simulink model "LH2Ship_Simulink_Winter"  (R2018b)
settings: Solver=VariableStepAuto  StartTime=0.0  StopTime=3600*24*7  FixedStep=0.1  MaxStep=0.5  MinStep=0.001  RelTol=1e-7  AbsTol=1e-7
values from neighbouring files (symbols this model uses):
  BoilerEff = 0.85    [PEMFC_Model.m]
  H2Consumption_kg = H2SupplyMolRate(:,1:iPmaxtot).*H2_kg_mol    [PEMFC_Model.m]
  H2Exhaust_kg = H2ExhaustMolRate(:,1:iPmaxtot).*H2_kg_mol    [PEMFC_Model.m]
  H2hhv = 141.7*10^6    (= 141700000)    [PEMFC_Model.m]
  H2lhv = 119.96*10^6    (= 119960000)    [PEMFC_Model.m]
  H2u = (0.05:0.1:0.95)    [PEMFC_Model.m]
  HeatStorageCapacity = 4.5e10    (= 45000000000)    [PEMFC_Model.m]
  HeatStorageEff = 0.9    [PEMFC_Model.m]
  HeatStorageIC = 1    [PEMFC_Model.m]
  i_FC = iCell(1,1:iPmaxtot)    [PEMFC_Model.m]
  Nstacks = 330    [PEMFC_Model.m]
  PowerElectronicsEff = 0.9    [PEMFC_Model.m]
  RecoveredHeat = NetHeatOut(:,1:iPmaxtot)    [PEMFC_Model.m]
  V_FC = Vout(:,1:iPmaxtot)    [PEMFC_Model.m]
undefined symbols (not defined in the file or in its folder): BatteryCapacity, BattInitialSOC, mass, Rt, v, VDCBus
libraries: fl_lib x14, nesl_utility x13, simulink x6, pe_lib x2
settings Model: SimulationMode=accelerator  Creator=age  LastModifiedBy=alber
settings SolverCC: InitialStep=0.001  MaxConsecutiveMinStep=2  ZeroCrossControl=DisableAll
settings DataIOCC: LimitDataPoints=on  MaxDataPoints=10000
settings OptimizationCC: LifeSpan=inf
settings DebuggingCC: AllowSymbolicDim=off  LibraryContextMissingDiagnostic=none  SFUnexpectedBacktrackingDiag=warning  SFNoUnconditionalDefaultTransitionDiag=warning  SFExecutionAtInitializationDiag=none
settings SFSimCC: SimUseLocalCustomCode=off
settings RTWCC: RTWUseLocalCustomCode=off
settings CodeAppCC: StateflowObjectComments=on
settings GRTTargetCC: TargetLangStandard=C89/C90 (ANSI)  GeneratePreprocessorConditionals=Disable all
settings ConfigComp: CovMetricSettings=dw  CovHtmlReporting=on  CovSaveCumulativeToWorkspaceVar=on  CovSaveSingleToWorkspaceVar=on  CovExternalEMLEnable=off  CovSFcnEnable=off
settings SimscapeCC: SimscapeLogLimitData=off  SimscapeLogDataHistory=10000

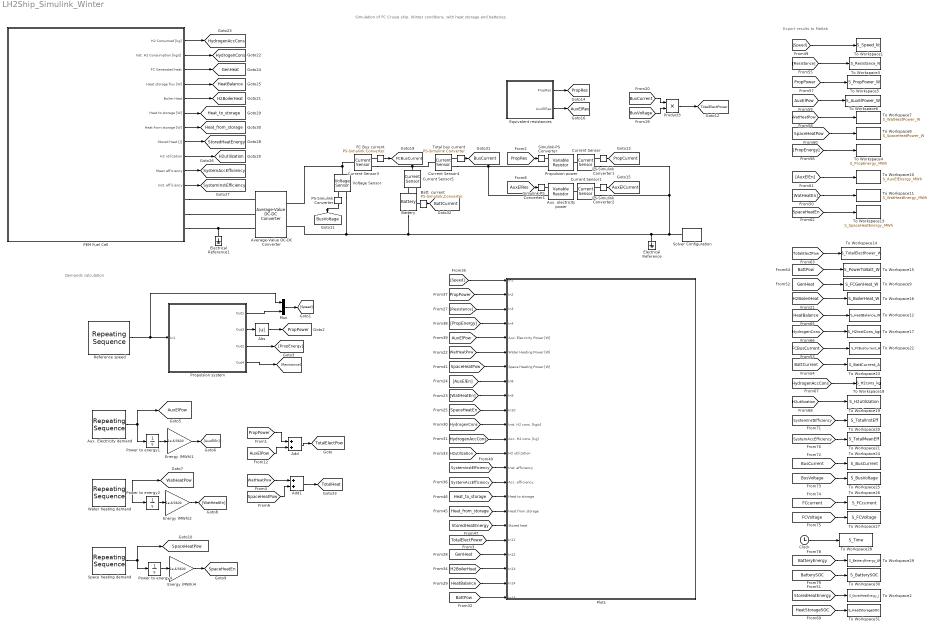
== system LH2Ship_Simulink_Winter ==
  note: Demands calculation
  note: Export results to Matlab
  note: Simulation of FC Cruise ship.
      | Winter conditions, with heat storage and batteries.
  Abs : Abs
  Add : Sum
  Add1 : Sum
  Aux. Electricity demand : simulink/Sources/Repeating Sequence  rep_seq_t=AuxElectProfile.t  rep_seq_y=AuxElectProfile.Elect  mask(Repeating table){}
      mask Display: image('RefSpeed.PNG');
  Aux. electricity power : fl_lib/Electrical/Electrical Elements/Variable Resistor  Rmin=2.8571e-4 Ohm  i_specify=off  i_priority=None  i=0 A  i_nominal_specify=off  i_nominal_unit=A  i_nominal_value=1  v_specify=off  v_priority=None  v=0 V  v_nominal_specify=off  v_nominal_unit=V  v_nominal_value=1
  Average-Value DC-DC Converter : pe_lib/Semiconductors/Average-Value DC-DC Converter  converter_type=3
      settings: SourceProductName=Simscape Power Systems  SourceProductBaseCode=PS
  Batt. current : nesl_utility/PS-Simulink Converter  PhysicalDomain=network_engine_domain  SubClassName=ps_output  LeftPortType=input  RightPortType=output  PseudoPeriodic=off  Frequencies=[]  Unit=1  AffineConversion=off
  Battery : pe_lib/Sources/Battery  Vnom=100 V  R1=0.00016667 Ohm  prm_AH=1  AH=6000 hr*A  V1=75 V  AH1=5426.087 hr*A  prm_R2=1  R2=2000 Ohm  prm_dyn=1  Rp1=0.0005 Ohm  tau1=10 s  Rp2=0.005 Ohm  tau2=30 s  Rp3=0.005 Ohm  tau3=30 s  Rp4=0.005 Ohm  tau4=30 s  Rp5=0.005 Ohm  tau5=30 s  prm_fade=1  N_fade=100  AH_fade=45 hr*A  R1_fade=2.02 Ohm  V1_fade=10.35 V  i_specify=on  i_priority=Low  i=0 A  i_nominal_specify=off  i_nominal_unit=A  i_nominal_value=1  v_specify=on  v_priority=None  v=100 V  v_nominal_specify=off  v_nominal_unit=V  v_nominal_value=1  charge_specify=on  charge_priority=High  charge=3000 hr*A  charge_nominal_specify=off  charge_nominal_unit=hr*A  charge_nominal_value=1  num_cycles_specify=on  num_cycles_priority=None  num_cycles=0  num_cycles_nominal_specify=off  num_cycles_nominal_unit=1  num_cycles_nominal_value=1  thermal_mass=30000 J/K  Tmeas=298.15 K  Vnom_T2=12 V  R1_T2=2.2 Ohm  V1_T2=11.4 V  R2_T2=2200 Ohm  Rp1_T2=0.005 Ohm  tau1_T2=30 s  Rp2_T2=0.005 Ohm  tau2_T2=30 s  Rp3_T2=0.005 Ohm  tau3_T2=30 s  Rp4_T2=0.005 Ohm  tau4_T2=30 s  Rp5_T2=0.005 Ohm  tau5_T2=30 s  Tmeas2=273.15 K  temperature_specify=off  temperature_priority=High  temperature=298.15 K  temperature_nominal_specify=off  temperature_nominal_unit=K  temperature_nominal_value=1
      settings: SourceProductName=Simscape Power Systems  SourceProductBaseCode=PS
  Clock : Clock
  Current Sensor{,1,3..5} (5 alike) : fl_lib/Electrical/Electrical Sensors/Current Sensor
  Electrical Reference : fl_lib/Electrical/Electrical Elements/Electrical Reference
      settings: SourceProductName=Foundation Library
  Electrical Reference1 : fl_lib/Electrical/Electrical Elements/Electrical Reference
      settings: SourceProductName=Foundation Library
  Energy (MWh)1 : Gain  Gain=1e-6/3600
  Energy (MWh)2 : Gain  Gain=1e-6/3600
  Energy (MWh)4 : Gain  Gain=1e-6/3600
  Equivalent resistances : Subsystem
  FC Bus current : nesl_utility/PS-Simulink Converter  PhysicalDomain=network_engine_domain  SubClassName=ps_output  LeftPortType=input  RightPortType=output  PseudoPeriodic=off  Frequencies=[]  Unit=1  AffineConversion=off
  Mux : Mux  Inputs=2
  PEM Fuel Cell : Subsystem
  PS-Simulink Converter : nesl_utility/PS-Simulink Converter  PhysicalDomain=network_engine_domain  SubClassName=ps_output  LeftPortType=input  RightPortType=output  PseudoPeriodic=off  Frequencies=[]  Unit=1  AffineConversion=off
  PS-Simulink Converter1 : nesl_utility/PS-Simulink Converter  PhysicalDomain=network_engine_domain  SubClassName=ps_output  LeftPortType=input  RightPortType=output  PseudoPeriodic=off  Frequencies=[]  Unit=1  AffineConversion=off
  PS-Simulink Converter2 : nesl_utility/PS-Simulink Converter  PhysicalDomain=network_engine_domain  SubClassName=ps_output  LeftPortType=input  RightPortType=output  PseudoPeriodic=off  Frequencies=[]  Unit=1  AffineConversion=off
  Plots : Subsystem
  Power to energy1 : Integrator  LowerSaturationLimit=0
  Power to energy2 : Integrator  LowerSaturationLimit=0
  Power to energy4 : Integrator  LowerSaturationLimit=0
  Product3 : Product
  Propulsion power : fl_lib/Electrical/Electrical Elements/Variable Resistor  Rmin=2.8571e-4 Ohm  i_specify=off  i_priority=None  i=0 A  i_nominal_specify=off  i_nominal_unit=A  i_nominal_value=1  v_specify=off  v_priority=None  v=0 V  v_nominal_specify=off  v_nominal_unit=V  v_nominal_value=1
  Propulsion system : Subsystem
  Reference speed : simulink/Sources/Repeating Sequence  rep_seq_t=SpeedProfile.Time  rep_seq_y=SpeedProfile.Speed  mask(Repeating table){}
      mask Display: image('RefSpeed.PNG');
  Simulink-PS Converter : nesl_utility/Simulink-PS Converter  PhysicalDomain=network_engine_domain  SubClassName=ps_input  LeftPortType=input  RightPortType=output  PseudoPeriodic=off  Frequencies=[]  NoiseDistribution=none  NoiseParameters=[]  Unit=1  AffineConversion=off  FilteringAndDerivatives=provide  SimscapeFilterOrder=1  InputFilterTimeConstant=0.001  UdotUserProvided=0
  Simulink-PS Converter1 : nesl_utility/Simulink-PS Converter  PhysicalDomain=network_engine_domain  SubClassName=ps_input  LeftPortType=input  RightPortType=output  PseudoPeriodic=off  Frequencies=[]  NoiseDistribution=none  NoiseParameters=[]  Unit=1  AffineConversion=off  FilteringAndDerivatives=provide  SimscapeFilterOrder=1  InputFilterTimeConstant=0.001  UdotUserProvided=0
  Solver Configuration : nesl_utility/Solver Configuration  PhysicalDomain=network_engine_domain  SubClassName=solver  LeftPortType=input  RightPortType=generic  Tones=[]  Harmonics=[]  SimulateNoise=off  Profile=off  UseLocalSampling=off  EnableSwitchedLinearOptims=on  FrequencyDomain=off  UseCCode=off  RelTol=0.001  AbsTol=1e-06  MinStep=1e-09  ToWorkspace=off  RevertToSquareIcSolve=off  NumHomotopyIterations=100  PhasorMode=off  PhasorModeNumHarmonics=1  DoDC=on  ResidualTolerance=1e-09  UseLocalSolver=off  LocalSolverChoice=NE_BACKWARD_EULER_ADVANCER  LocalSolverSampleTime=0.001  DoFixedCost=off  MaxNonlinIter=3  MaxModeIter=2  LinearAlgebra=auto  EquationFormulation=NE_TIME_EF  DelaysMemoryBudget=1024  AutomaticFiltering=on  FilteringTimeConstant=0.001  PartitionStorageMethod=AS_NEEDED  PartitionMemoryBudget=1024
  Space heating demand : simulink/Sources/Repeating Sequence  rep_seq_t=SpaceHeatingProfile_Winter.t  rep_seq_y=SpaceHeatingProfile_Winter.Heat  mask(Repeating table){}
      mask Display: image('RefSpeed.PNG');
  To Workspace1 : ToWorkspace  VariableName=S_Speed_kt  SampleTime=30
  To Workspace10 : ToWorkspace  VariableName=S_AuxElEnergy_MWh  SampleTime=30
  To Workspace11 : ToWorkspace  VariableName=S_WatHeatEnergy_MWh  SampleTime=30
  To Workspace12 : ToWorkspace  VariableName=S_HeatBalance_W  SampleTime=30
  To Workspace13 : ToWorkspace  VariableName=S_SpaceHeatEnergy_MWh  SampleTime=30
  To Workspace14 : ToWorkspace  VariableName=S_TotalElectPower_W  SampleTime=30
  To Workspace15 : ToWorkspace  VariableName=S_PowerToBatt_W  SampleTime=30
  To Workspace16 : ToWorkspace  VariableName=S_BoilerHeat_W  SampleTime=30
  To Workspace17 : ToWorkspace  VariableName=S_H2instCons_kgs  SampleTime=30
  To Workspace18 : ToWorkspace  VariableName=S_H2cons_kg  SampleTime=30
  To Workspace19 : ToWorkspace  VariableName=S_H2utilization  SampleTime=30
  To Workspace2 : ToWorkspace  VariableName=S_StoredHeatEnergy_J  SampleTime=30
  To Workspace20 : ToWorkspace  VariableName=S_TotalInstEff  SampleTime=30
  To Workspace21 : ToWorkspace  VariableName=S_TotalMeanEff  SampleTime=30
  To Workspace22 : ToWorkspace  VariableName=S_FCBusCurrent_A  SampleTime=30
  To Workspace23 : ToWorkspace  VariableName=S_BattCurrent_A  SampleTime=30
  To Workspace24 : ToWorkspace  VariableName=S_BusCurrent  SampleTime=30
  To Workspace25 : ToWorkspace  VariableName=S_BusVoltage  SampleTime=30
  To Workspace26 : ToWorkspace  VariableName=S_FCcurrent  SampleTime=30
  To Workspace27 : ToWorkspace  VariableName=S_FCVoltage  SampleTime=30
  To Workspace28 : ToWorkspace  VariableName=S_Time  SampleTime=30
  To Workspace29 : ToWorkspace  VariableName=S_BatteryEnergy_Ah  SampleTime=30
  To Workspace3 : ToWorkspace  VariableName=S_Resistance_N  SampleTime=30
  To Workspace30 : ToWorkspace  VariableName=S_BatterySOC  SampleTime=30
  To Workspace31 : ToWorkspace  VariableName=S_HeatStorageSOC  SampleTime=30
  To Workspace4 : ToWorkspace  VariableName=S_PropEnergy_MWh  SampleTime=30
  To Workspace5 : ToWorkspace  VariableName=S_PropPower_W  SampleTime=30
  To Workspace6 : ToWorkspace  VariableName=S_AuxElPower_W  SampleTime=30
  To Workspace7 : ToWorkspace  VariableName=S_WatHeatPower_W  SampleTime=30
  To Workspace8 : ToWorkspace  VariableName=S_SpaceHeatPower_W  SampleTime=30
  To Workspace9 : ToWorkspace  VariableName=S_FCGenHeat_W  SampleTime=30
  Total bus current : nesl_utility/PS-Simulink Converter  PhysicalDomain=network_engine_domain  SubClassName=ps_output  LeftPortType=input  RightPortType=output  PseudoPeriodic=off  Frequencies=[]  Unit=1  AffineConversion=off
  Voltage Sensor : fl_lib/Electrical/Electrical Sensors/Voltage Sensor
  Water heating demand : simulink/Sources/Repeating Sequence  rep_seq_t=WaterHeatingProfile.t  rep_seq_y=WaterHeatingProfile.Heat  mask(Repeating table){}
      mask Display: image('RefSpeed.PNG');
  tag scope: AuxElCurrent=global, AuxElPow=global, AuxElRes=global, BattCurrent=global, BusCurrent=global, BusVoltage=global, FCBusCurrent=global, GenHeat=global, H2BoilerHeat=global, H2utilization=global, HeatBalance=global, Heat_from_storage=global, Heat_to_storage=global, HydrogenAccCons=global, HydrogenCons=global, PropCurrent=global, PropPower=global, PropRes=global, SpaceHeatEn=global, SpaceHeatPow=global, StoredHeatEnergy=global, SystemAccEfficiency=global, SystemInstEfficiency=global, TotalElectPow=global, TotalElectPower=global, TotalHeat=global, WatHeatPow=global
  wires:
  Power to energy1/1 -> Energy (MWh)1/1
  Propulsion system/4(Out4) -> [Resistance]
  Water heating demand/1 -> [WatHeatPow], Power to energy2/1
  Mux/1 -> [Speed]
  Propulsion system/3(Out2) -> [PropEnergy]
  Power to energy2/1 -> Energy (MWh)2/1
  [PropPower] -> Add/1
  [AuxElPow] -> Add/2
  Propulsion system/1(Out1) -> Mux/2
  Reference speed/1 -> Mux/1, Propulsion system/1(In1)
  Energy (MWh)2/1 -> [WatHeatEn]
  Add/1 -> [TotalElectPow]
  Aux. Electricity demand/1 -> [AuxElPow], Power to energy1/1
  Energy (MWh)1/1 -> [AuxElEn]
  PS-Simulink Converter/1 -> [BusVoltage]
  PS-Simulink Converter1/1 -> [PropCurrent]
  Equivalent resistances/1(PropRes) -> [PropRes]
  [PropRes] -> Simulink-PS Converter/1
  [AuxElRes] -> Simulink-PS Converter1/1
  PS-Simulink Converter2/1 -> [AuxElCurrent]
  Equivalent resistances/2(AuxElRes) -> [AuxElRes]
  FC Bus current/1 -> [FCBusCurrent]
  PEM Fuel Cell/9(H2 utilization) -> [H2utilization]
  PEM Fuel Cell/7(Heat from storage [W]) -> [Heat_from_storage]
  PEM Fuel Cell/8(Stored Heat [J]) -> [StoredHeatEnergy]
  PEM Fuel Cell/6(Heat to storage [W]) -> [Heat_to_storage]
  PEM Fuel Cell/5(Boiler Heat) -> [H2BoilerHeat]
  PEM Fuel Cell/4(Heat storage flux [W]) -> [HeatBalance]
  PEM Fuel Cell/3(FC Generated heat) -> [GenHeat]
  PEM Fuel Cell/2(Inst. H2 Consumption [kg/s]) -> [HydrogenCons]
  PEM Fuel Cell/1(H2 Consumed [kg]) -> [HydrogenAccCons]
  [Speed] -> Plots/1(In1)
  [BattPow] -> Plots/23(In23)
  [GenHeat] -> Plots/20(In12)
  [WatHeatEn] -> Plots/9(In9)
  [Heat_to_storage] -> Plots/16(Heat to storage)
  [SystemAccEfficiency] -> Plots/15(Acc. efficiency)
  [H2utilization] -> Plots/13(H2 utilization)
  [SpaceHeatPow] -> Plots/7(Space Heating Power [W])
  [AuxElPow] -> Plots/5(Aux. Elecricity Power [W])
  [StoredHeatEnergy] -> Plots/18(Stored heat)
  [SystemInstEfficiency] -> Plots/14(Inst. efficiency)
  [AuxElEn] -> Plots/8(In8)
  [Heat_from_storage] -> Plots/17(Heat from storage)
  [HydrogenCons] -> Plots/11(Inst. H2 cons. [kg/s])
  [HeatBalance] -> Plots/22(In14)
  [PropPower] -> Plots/2(In2)
  [PropEnergy] -> Plots/4(In4)
  [HydrogenAccCons] -> Plots/12(Acc. H2 cons. [kg])
  [H2BoilerHeat] -> Plots/21(In13)
  [Resistance] -> Plots/3(In3)
  [WatHeatPow] -> Plots/6(Water Heating Power [W])
  [SpaceHeatEn] -> Plots/10(In10)
  PEM Fuel Cell/10(Mean efficiency) -> [SystemAccEfficiency]
  PEM Fuel Cell/11(Inst. efficiency) -> [SystemInstEfficiency]
  Total bus current/1 -> [BusCurrent]
  Batt. current/1 -> [BattCurrent]
  [WatHeatEn] -> To Workspace11/1
  [Resistance] -> To Workspace3/1
  [GenHeat] -> To Workspace9/1
  [Speed] -> To Workspace1/1
  [SystemAccEfficiency] -> To Workspace21/1
  [WatHeatPow] -> To Workspace7/1
  [PropPower] -> To Workspace5/1
  [HydrogenCons] -> To Workspace17/1
  [FCBusCurrent] -> To Workspace22/1
  [BattPow] -> To Workspace15/1
  [BattCurrent] -> To Workspace23/1
  [SystemInstEfficiency] -> To Workspace20/1
  [HydrogenAccCons] -> To Workspace18/1
  [H2utilization] -> To Workspace19/1
  [PropEnergy] -> To Workspace4/1
  [H2BoilerHeat] -> To Workspace16/1
  [HeatBalance] -> To Workspace12/1
  [SpaceHeatPow] -> To Workspace8/1
  [AuxElPow] -> To Workspace6/1
  [SpaceHeatEn] -> To Workspace13/1
  [AuxElEn] -> To Workspace10/1
  [TotalElectPow] -> To Workspace14/1
  [BusCurrent] -> To Workspace24/1
  [BusVoltage] -> To Workspace25/1
  [FCcurrent] -> To Workspace26/1
  [FCVoltage] -> To Workspace27/1
  Clock/1 -> To Workspace28/1
  [BatterySOC] -> To Workspace30/1
  [BatteryEnergy] -> To Workspace29/1
  Propulsion system/2(Out3) -> Abs/1
  Abs/1 -> [PropPower]
  [HeatStorageSOC] -> To Workspace31/1
  [StoredHeatEnergy] -> To Workspace2/1
  Product3/1 -> [TotalElectPower]
  [BusVoltage] -> Product3/2
  [BusCurrent] -> Product3/1
  [TotalElectPower] -> Plots/19(In11)
  Energy (MWh)4/1 -> [SpaceHeatEn]
  Space heating demand/1 -> Power to energy4/1, [SpaceHeatPow]
  Power to energy4/1 -> Energy (MWh)4/1
  Add1/1 -> [TotalHeat]
  [SpaceHeatPow] -> Add1/2
  [WatHeatPow] -> Add1/1
  connections:
  Simulink-PS Converter/RConn1 -- Propulsion power/LConn1
  Current Sensor/LConn1 -- Propulsion power/RConn1
  Current Sensor/RConn2 -- Current Sensor1/RConn2 -- Voltage Sensor/RConn2 -- Average-Value DC-DC Converter/RConn2 -- Battery/RConn1 -- Electrical Reference/LConn1 -- Solver Configuration/RConn1
  PS-Simulink Converter/LConn1 -- Voltage Sensor/RConn1
  Current Sensor/RConn1 -- PS-Simulink Converter1/LConn1
  Aux. electricity power/LConn2 -- Current Sensor4/RConn2 -- Propulsion power/LConn2
  PEM Fuel Cell/RConn1 -- Average-Value DC-DC Converter/LConn1
  PEM Fuel Cell/RConn2 -- Average-Value DC-DC Converter/LConn2
  PEM Fuel Cell/RConn3 -- Electrical Reference1/LConn1 -- Average-Value DC-DC Converter/LConn3
  Current Sensor1/LConn1 -- Aux. electricity power/RConn1
  Current Sensor1/RConn1 -- PS-Simulink Converter2/LConn1
  Simulink-PS Converter1/RConn1 -- Aux. electricity power/LConn1
  Current Sensor3/RConn1 -- FC Bus current/LConn1
  Voltage Sensor/LConn1 -- Current Sensor3/LConn1 -- Average-Value DC-DC Converter/RConn1
  Current Sensor3/RConn2 -- Current Sensor4/LConn1 -- Current Sensor5/LConn1
  Current Sensor4/RConn1 -- Total bus current/LConn1
  Current Sensor5/RConn1 -- Batt. current/LConn1
  Battery/LConn1 -- Current Sensor5/RConn2

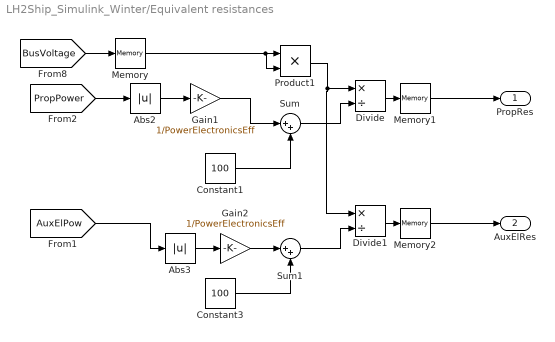
== system LH2Ship_Simulink_Winter/Equivalent resistances ==
  Abs2 : Abs
  Abs3 : Abs
  Constant1 : Constant  Value=100
  Constant3 : Constant  Value=100
  Divide : Product  Inputs=*/
  Divide1 : Product  Inputs=*/
  Gain1 : Gain  Gain=1/PowerElectronicsEff
  Gain2 : Gain  Gain=1/PowerElectronicsEff
  Memory : Memory  InitialCondition=100
  Memory1 : Memory  InitialCondition=0.0005
  Memory2 : Memory  InitialCondition=0.0005
  Product1 : Product
  Sum : Sum  Inputs=|++
  Sum1 : Sum  Inputs=|++
  PropRes : Outport
  AuxElRes : Outport  Port=2
  wires:
  Divide/1 -> Memory1/1
  Memory/1 -> Product1/2, Product1/1
  Constant1/1 -> Sum/2
  [BusVoltage] -> Memory/1
  Sum/1 -> Divide/2
  Memory1/1 -> PropRes/1
  [AuxElPow] -> Abs3/1
  Sum1/1 -> Divide1/2
  Constant3/1 -> Sum1/2
  Divide1/1 -> Memory2/1
  Memory2/1 -> AuxElRes/1
  Product1/1 -> Divide1/1, Divide/1
  [PropPower] -> Abs2/1
  Abs2/1 -> Gain1/1
  Gain1/1 -> Sum/1
  Abs3/1 -> Gain2/1
  Gain2/1 -> Sum1/1

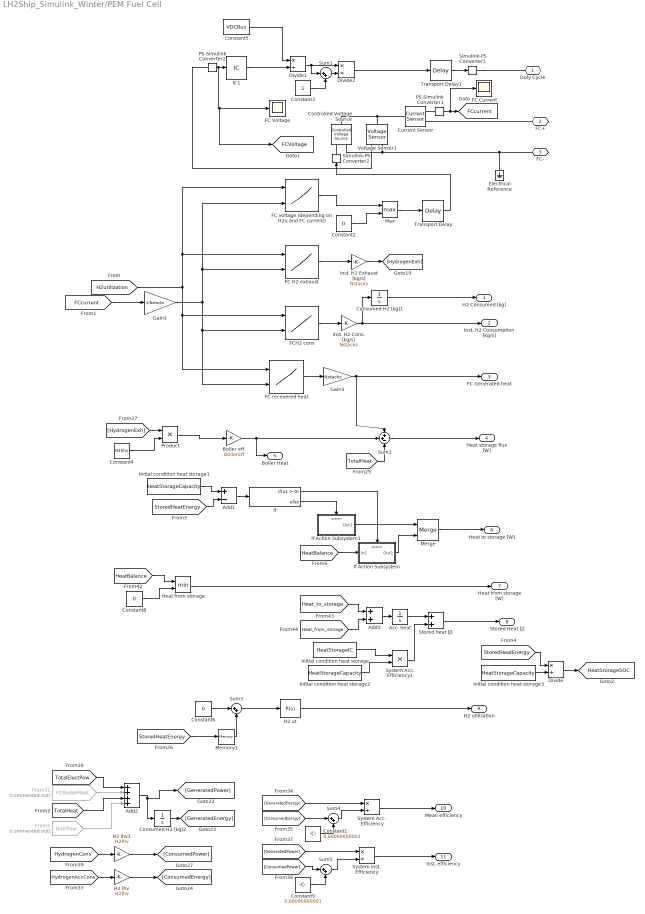
== system LH2Ship_Simulink_Winter/PEM Fuel Cell ==
  Acc. heat : Integrator  InitialCondition=0.00000000001
  Add1 : Sum  Inputs=+-
  Add2 : Sum  Inputs=++++
  Add3 : Sum
  Boiler eff. : Gain  Gain=BoilerEff
  Constant1 : Constant  Value=0.00000000001
  Constant2 : Constant  Value=0
  Constant3 : Constant
  Constant4 : Constant  Value=H2hhv
  Constant5 : Constant  Value=VDCBus
  Constant6 : Constant  Value=0
  Constant8 : Constant  Value=0
  Constant9 : Constant  Value=0.00000000001
  Consumed H2 [kg]1 : Integrator
  Consumed H2 [kg]2 : Integrator  InitialCondition=0.00000000001
  Controlled Voltage Source : fl_lib/Electrical/Electrical Sources/Controlled Voltage Source
  Current Sensor : fl_lib/Electrical/Electrical Sensors/Current Sensor
  Divide : Product  Inputs=*/
  Divide1 : Product  Inputs=*/
  Divide2 : Product  Inputs=*/
  Electrical Reference : fl_lib/Electrical/Electrical Elements/Electrical Reference
      settings: SourceProductName=Foundation Library
  FC Current : Scope
  FC H2 exhaust : Lookup_n-D  BreakpointsForDimension1=H2u  BreakpointsForDimension2=i_FC  Table=H2Exhaust_kg  InternalRulePriority=Speed  RndMeth=Simplest  InputSameDT=on
  FC Voltage : Scope
  FC recovered heat : Lookup_n-D  BreakpointsForDimension1=H2u  BreakpointsForDimension2=i_FC  Table=RecoveredHeat  InternalRulePriority=Speed  RndMeth=Simplest  InputSameDT=on
  FC voltage (depending on H2u and FC current) : Lookup_n-D  BreakpointsForDimension1=H2u  BreakpointsForDimension2=i_FC  Table=V_FC  InternalRulePriority=Speed  RndMeth=Simplest  InputSameDT=on
  FCH2 cons : Lookup_n-D  BreakpointsForDimension1=H2u  BreakpointsForDimension2=i_FC  Table=H2Consumption_kg  InternalRulePriority=Speed  RndMeth=Simplest  InputSameDT=on
  From31 : From  Commented=on  GotoTag=H2BoilerHeat
  From5 : From  Commented=on  GotoTag=BattPow  TagVisibility=global
  Gain1 : Gain  Gain=1/Nstacks
  Gain3 : Gain  Gain=Nstacks
  H2 lhv : Gain  Gain=H2lhv
  H2 lhv1 : Gain  Gain=H2lhv
  H2 ut : simulink/Continuous/PID Controller  Controller=P  Form=Parallel  TimeDomain=Continuous-time  SampleTime=-1  IntegratorMethod=Forward Euler  FilterMethod=Forward Euler  ControllerParametersSource=internal  P=5.19805668367271e-09  I=5.74544625203428e-08  D=7000000  UseFilter=on  N=0.01  TunerSelectOption=Transfer Function Based (PID Tuner App)  InitialConditionSource=internal  InitialConditionForIntegrator=0.95  InitialConditionForFilter=0.1  DifferentiatorICPrevScaledInput=0  ExternalReset=none  TrackingMode=off  Kt=1  LimitOutput=on  UpperSaturationLimit=0.95  LowerSaturationLimit=0.05  LinearizeAsGain=off  AntiWindupMode=clamping  Kb=1  POutMin=[]  POutMax=[]  IOutMin=[]  IOutMax=[]  DOutMin=[]  DOutMax=[]  NOutMin=[]  NOutMax=[]  SumOutMin=[]  SumOutMax=[]  SaturationOutMin=[]  SaturationOutMax=[]  PParamMin=[]  PParamMax=[]  IParamMin=[]  IParamMax=[]  DParamMin=[]  DParamMax=[]  NParamMin=[]  NParamMax=[]  KbParamMin=[]  KbParamMax=[]  KtParamMin=[]  KtParamMax=[]  KbOutMin=[]  KbOutMax=[]  KtOutMin=[]  KtOutMax=[]  IntegratorOutMin=[]  IntegratorOutMax=[]  FilterOutMin=[]  FilterOutMax=[]  SumI1OutMin=[]  SumI1OutMax=[]  SumI2OutMin=[]  SumI2OutMax=[]  SumI3OutMin=[]  SumI3OutMax=[]  SumI4OutMin=[]  SumI4OutMax=[]  SumDOutMin=[]  SumDOutMax=[]  DifferentiatorOutMin=[]  DifferentiatorOutMax=[]  FilterDiffOutCoefMin=[]  FilterDiffOutCoefMax=[]  ReciprocalOutMin=[]  ReciprocalOutMax=[]  SumDenOutMin=[]  SumDenOutMax=[]  SumNumOutMin=[]  SumNumOutMax=[]  DivideOutMin=[]  DivideOutMax=[]  IntegratorContinuousStateAttributes=''  IntegratorStateMustResolveToSignalObject=off  IntegratorRTWStateStorageClass=Auto  FilterContinuousStateAttributes=''  FilterStateMustResolveToSignalObject=off  FilterRTWStateStorageClass=Auto  ParallelPVariant=InternalParameters  IdealPVariant=Disabled  IVariant=Disabled  DVariant=Disabled  IntegratorVariant=Disabled  SatVariant=Enabled  AWVariant=Disabled  PCopyVariant=Disabled  TRVariant=Disabled  FdbkBlocksVariant=Forward  IdealPFdbkVariant=Disabled  SatFdbkVariant=Disabled  DerivativeFilterVariant=Disabled  NVariant=Disabled  NCopyVariant=Disabled_SignalSpec  FilterICVariant=Disabled  IntegratorICVariant=Disabled  ExternalResetVariant=Disabled  TRSumVariant=Passthrough  SumFdbkVariant=Disabled  SumVariant=Passthrough_P
  "Heat from storage " : MinMax  Inputs=2
  IC1 : InitialCondition  Value=110
  If : If
  If Action Subsystem : Subsystem  TreatAsAtomicUnit=on
  If Action Subsystem1 : Subsystem  TreatAsAtomicUnit=on
  Initial condition heat storage : Constant  Value=HeatStorageIC
  Initial condition heat storage1 : Constant  Value=HeatStorageCapacity
  Initial condition heat storage2 : Constant  Value=HeatStorageCapacity
  Initial condition heat storage3 : Constant  Value=HeatStorageCapacity
  Inst. H2 Cons. [kg/s] : Gain  Gain=Nstacks
  Inst. H2 Exhaust [kg/s] : Gain  Gain=Nstacks
  Max : MinMax  Function=max  Inputs=2
  Memory1 : Memory  InitialCondition=HeatStorageCapacity*HeatStorageIC
  Merge : Merge
  PS-Simulink Converter1 : nesl_utility/PS-Simulink Converter  PhysicalDomain=network_engine_domain  SubClassName=ps_output  LeftPortType=input  RightPortType=output  PseudoPeriodic=off  Frequencies=[]  Unit=1  AffineConversion=off
  PS-Simulink Converter2 : nesl_utility/PS-Simulink Converter  PhysicalDomain=network_engine_domain  SubClassName=ps_output  LeftPortType=input  RightPortType=output  PseudoPeriodic=off  Frequencies=[]  Unit=1  AffineConversion=off
  Product : Product
  Simulink-PS Converter1 : nesl_utility/Simulink-PS Converter  PhysicalDomain=network_engine_domain  SubClassName=ps_input  LeftPortType=input  RightPortType=output  PseudoPeriodic=off  Frequencies=[]  NoiseDistribution=none  NoiseParameters=[]  Unit=1  AffineConversion=off  FilteringAndDerivatives=provide  SimscapeFilterOrder=1  InputFilterTimeConstant=0.001  UdotUserProvided=0
  Simulink-PS Converter2 : nesl_utility/Simulink-PS Converter  PhysicalDomain=network_engine_domain  SubClassName=ps_input  LeftPortType=input  RightPortType=output  PseudoPeriodic=off  Frequencies=[]  NoiseDistribution=none  NoiseParameters=[]  Unit=1  AffineConversion=off  FilteringAndDerivatives=provide  SimscapeFilterOrder=1  InputFilterTimeConstant=0.001  UdotUserProvided=0
  Stored heat [J] : Sum
  Sum{1,3..5} (4 alike) : Sum  Inputs=|++
  Sum2 : Sum  Inputs=++-
  System Acc. Efficiency : Product  Inputs=*/
  System Acc. Efficiency1 : Product  Inputs=**
  System inst. Efficiency : Product  Inputs=*/
  Transport Delay : TransportDelay  DelayTime=60  InitialOutput=110
  Transport Delay1 : TransportDelay  DelayTime=30  InitialOutput=0.4762
  Voltage Sensor1 : fl_lib/Electrical/Electrical Sensors/Voltage Sensor
  Duty Cycle : PMIOPort  Side=Right
  FC+ : PMIOPort  Port=2  Side=Right
  FC- : PMIOPort  Port=3  Side=Right
  H2 Consumed [kg] : Outport
  Inst. H2 Consumption [kg/s] : Outport  Port=2
  FC Generated heat : Outport  Port=3
  Heat storage flux [W] : Outport  Port=4
  Boiler Heat : Outport  Port=5
  Heat to storage [W] : Outport  Port=6
  Heat from storage [W] : Outport  Port=7
  Stored Heat [J] : Outport  Port=8
  H2 utilization : Outport  Port=9
  Mean efficiency : Outport  Port=10
  Inst. efficiency : Outport  Port=11
  tag scope: FCVoltage=global, FCcurrent=global, HeatStorageSOC=global
  wires:
  Constant3/1 -> Sum1/2
  Divide1/1 -> Sum1/1, Divide2/1
  Constant5/1 -> Divide1/1
  PS-Simulink Converter2/1 -> [FCVoltage], FC Voltage/1, IC1/1
  Sum1/1 -> Divide2/2
  FC voltage (depending on H2u and FC current)/1 -> Max/1
  [H2utilization] -> FC recovered heat/1, FCH2 cons/1, FC H2 exhaust/1, FC voltage (depending on H2u and FC current)/1
  Gain1/1 -> FC H2 exhaust/2, FC voltage (depending on H2u and FC current)/2, FCH2 cons/2, FC recovered heat/2
  PS-Simulink Converter1/1 -> FC Current/1, [FCcurrent]
  Constant2/1 -> Max/2
  FC H2 exhaust/1 -> Inst. H2 Exhaust [kg/s]/1
  FCH2 cons/1 -> Inst. H2 Cons. [kg/s]/1
  Constant4/1 -> Product/2
  Sum2/1 -> Heat storage flux [W]/1
  Product/1 -> Boiler eff./1
  Inst. H2 Cons. [kg/s]/1 -> Inst. H2 Consumption [kg/s]/1, Consumed H2 [kg]1/1
  [HydrogenExh] -> Product/1
  Inst. H2 Exhaust [kg/s]/1 -> [HydrogenExh]
  Consumed H2 [kg]1/1 -> H2 Consumed [kg]/1
  Boiler eff./1 -> Boiler Heat/1, Sum2/2
  Gain3/1 -> Sum2/1, FC Generated heat/1
  [TotalHeat] -> Sum2/3
  FC recovered heat/1 -> Gain3/1
  Constant8/1 -> "Heat from storage "/2
  [Heat_to_storage] -> Add3/1
  "Heat from storage "/1 -> Heat from storage [W]/1
  [Heat_from_storage] -> Add3/2
  [HeatBalance] -> "Heat from storage "/1
  Acc. heat/1 -> Stored heat [J]/1
  Add3/1 -> Acc. heat/1
  Constant6/1 -> Sum3/1
  H2 ut/1 -> H2 utilization/1
  From5/1 -> Add2/4
  System Acc. Efficiency/1 -> Mean efficiency/1
  [TotalHeat] -> Add2/3
  [HydrogenAccCons] -> H2 lhv/1
  [TotalElectPow] -> Add2/1
  System inst. Efficiency/1 -> Inst. efficiency/1
  [GeneratedEnergy] -> System Acc. Efficiency/1
  Consumed H2 [kg]2/1 -> [GeneratedEnergy]
  H2 lhv1/1 -> [ConsumedPower]
  H2 lhv/1 -> [ConsumedEnergy]
  [ConsumedEnergy] -> Sum4/1
  From31/1 -> Add2/2
  Add2/1 -> Consumed H2 [kg]2/1, [GeneratedPower]
  [HydrogenCons] -> H2 lhv1/1
  [GeneratedPower] -> System inst. Efficiency/1
  [FCcurrent] -> Gain1/1
  [StoredHeatEnergy] -> Memory1/1
  Memory1/1 -> Sum3/2
  Sum3/1 -> H2 ut/1
  Constant1/1 -> Sum4/2
  Sum4/1 -> System Acc. Efficiency/2
  [ConsumedPower] -> Sum5/1
  Constant9/1 -> Sum5/2
  Sum5/1 -> System inst. Efficiency/2
  IC1/1 -> Divide1/2
  Max/1 -> Transport Delay/1
  Transport Delay/1 -> Simulink-PS Converter2/1
  Transport Delay1/1 -> Simulink-PS Converter1/1
  Divide2/1 -> Transport Delay1/1
  Add1/1 -> If/1
  Initial condition heat storage1/1 -> Add1/1
  [StoredHeatEnergy] -> Add1/2
  If/1 -> If Action Subsystem/Action
  [HeatBalance] -> If Action Subsystem/1(In1)
  If/2 -> If Action Subsystem1/Action
  If Action Subsystem/1(Out1) -> Merge/2
  If Action Subsystem1/1(Out1) -> Merge/1
  Merge/1 -> Heat to storage [W]/1
  Initial condition heat storage2/1 -> System Acc. Efficiency1/2
  Initial condition heat storage/1 -> System Acc. Efficiency1/1
  System Acc. Efficiency1/1 -> Stored heat [J]/2
  Stored heat [J]/1 -> Stored Heat [J]/1
  Initial condition heat storage3/1 -> Divide/2
  [StoredHeatEnergy] -> Divide/1
  Divide/1 -> [HeatStorageSOC]
  connections:
  Voltage Sensor1/RConn1 -- PS-Simulink Converter2/LConn1
  Voltage Sensor1/LConn1 -- Current Sensor/LConn1 -- Controlled Voltage Source/LConn1
  Simulink-PS Converter2/RConn1 -- Controlled Voltage Source/RConn1
  Controlled Voltage Source/RConn2 -- Electrical Reference/LConn1 -- FC-/RConn1 -- Voltage Sensor1/RConn2
  Simulink-PS Converter1/RConn1 -- Duty Cycle/RConn1
  PS-Simulink Converter1/LConn1 -- Current Sensor/RConn1
  FC+/RConn1 -- Current Sensor/RConn2

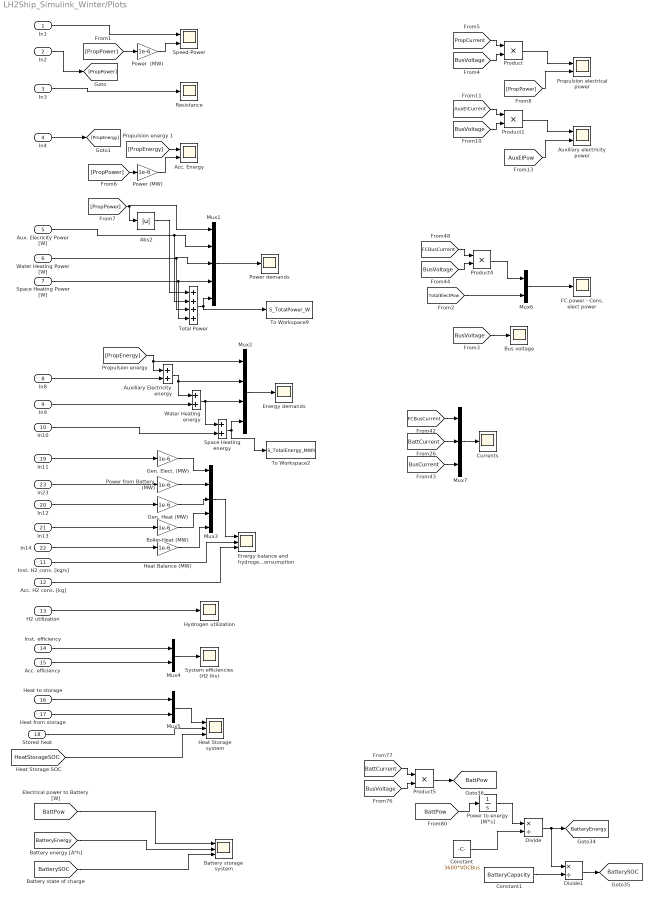
== system LH2Ship_Simulink_Winter/Plots ==
  In1 : Inport
  In2 : Inport  Port=2
  In3 : Inport  Port=3
  In4 : Inport  Port=4
  Aux. Elecricity Power [W] : Inport  Port=5
  Water Heating Power [W] : Inport  Port=6
  Space Heating Power [W] : Inport  Port=7
  In8 : Inport  Port=8
  In9 : Inport  Port=9
  In10 : Inport  Port=10
  Inst. H2 cons. [kg/s] : Inport  Port=11
  Acc. H2 cons. [kg] : Inport  Port=12
  H2 utilization : Inport  Port=13
  Inst. efficiency : Inport  Port=14
  Acc. efficiency : Inport  Port=15
  Heat to storage : Inport  Port=16
  Heat from storage : Inport  Port=17
  Stored heat : Inport  Port=18
  In11 : Inport  Port=19
  In12 : Inport  Port=20
  In13 : Inport  Port=21
  In14 : Inport  Port=22
  In23 : Inport  Port=23
  Abs2 : Abs
  Acc. Energy : Scope  NumInputPorts=2
  Auxiliary Electricity energy : Sum
  Auxiliary electricity power : Scope  NumInputPorts=2
  Battery storage system : Scope  NumInputPorts=3
  Boiler Heat (MW) : Gain  Gain=1e-6
  Bus voltage : Scope
  Constant : Constant  Value=3600*VDCBus
  Constant1 : Constant  Value=BatteryCapacity
  Currents : Scope
  Divide : Product  Inputs=*/
  Divide1 : Product  Inputs=*/
  Energy balance and hydrogen consumption : Scope  NumInputPorts=3
  Energy demands : Scope
  FC power - Cons. elect power : Scope
  Gen. Elect. (MW) : Gain  Gain=1e-6
  Gen. Heat (MW) : Gain  Gain=1e-6
  Heat Balance (MW) : Gain  Gain=1e-6
  Heat Storage system : Scope  NumInputPorts=3
  Hydrogen utilization : Scope
  Mux1 : Mux  Inputs=5
  Mux2 : Mux
  Mux3 : Mux  Inputs=5
  Mux4 : Mux  Inputs=2
  Mux5 : Mux  Inputs=2
  Mux6 : Mux  Inputs=2
  Mux7 : Mux  Inputs=3
  Power  (MW) : Gain  Gain=1e-6
  Power (MW) : Gain  Gain=1e-6
  Power demands : Scope
  Power from Battery (MW) : Gain  Gain=1e-6
  Power to energy [W*s] : Integrator  InitialCondition=BatteryCapacity*BattInitialSOC*VDCBus*3600  LowerSaturationLimit=0
  Product{,1,4..5} (4 alike) : Product
  Propulsion electrical power : Scope  NumInputPorts=2
  Resistance : Scope
  Space Heating energy : Sum
  Speed-Power : Scope  NumInputPorts=2
  System efficiencies (H2 lhv) : Scope
  To Workspace2 : ToWorkspace  VariableName=S_TotalEnergy_MWh  SampleTime=30
  To Workspace9 : ToWorkspace  VariableName=S_TotalPower_W  SampleTime=30
  Total Power : Sum  Inputs=++++
  Water Heating energy : Sum
  tag scope: BattPow=global, BatteryEnergy=global, BatterySOC=global
  wires:
  Mux4/1 -> System efficiencies (H2 lhv)/1
  Aux. Elecricity Power [W]/1 -> Mux1/2, Total Power/2
  Auxiliary Electricity energy/1 -> Water Heating energy/1, Mux2/2
  In9/1 -> Water Heating energy/2
  Acc. efficiency/1 -> Mux4/2
  Water Heating Power [W]/1 -> Mux1/3, Total Power/3
  Total Power/1 -> To Workspace9/1, Mux1/5
  Power  (MW)/1 -> Speed-Power/2
  Mux5/1 -> Heat Storage system/1
  [PropPower] -> Mux1/1, Abs2/1
  Abs2/1 -> Total Power/1
  [PropPower] -> Power (MW)/1
  [PropEnergy] -> Auxiliary Electricity energy/1, Mux2/1
  Mux2/1 -> Energy demands/1
  Water Heating energy/1 -> Mux2/3, Space Heating energy/1
  Space Heating energy/1 -> To Workspace2/1, Mux2/4
  Space Heating Power [W]/1 -> Total Power/4, Mux1/4
  Mux1/1 -> Power demands/1
  Power (MW)/1 -> Acc. Energy/2
  Stored heat/1 -> Heat Storage system/2
  Inst. efficiency/1 -> Mux4/1
  Acc. H2 cons. [kg]/1 -> Energy balance and hydrogen consumption/3
  Heat to storage/1 -> Mux5/1
  Heat from storage/1 -> Mux5/2
  In8/1 -> Auxiliary Electricity energy/2
  In3/1 -> Resistance/1
  Inst. H2 cons. [kg/s]/1 -> Energy balance and hydrogen consumption/2
  H2 utilization/1 -> Hydrogen utilization/1
  In10/1 -> Space Heating energy/2
  In1/1 -> Speed-Power/1
  In2/1 -> [PropPower]
  [PropPower] -> Power  (MW)/1
  In4/1 -> [PropEnergy]
  [PropEnergy] -> Acc. Energy/1
  In23/1 -> Power from Battery (MW)/1
  Gen. Heat (MW)/1 -> Mux3/3
  Mux3/1 -> Energy balance and hydrogen consumption/1
  Boiler Heat (MW)/1 -> Mux3/4
  In14/1 -> Heat Balance (MW)/1
  Power from Battery (MW)/1 -> Mux3/2
  In11/1 -> Gen. Elect. (MW)/1
  In13/1 -> Boiler Heat (MW)/1
  Gen. Elect. (MW)/1 -> Mux3/1
  Heat Balance (MW)/1 -> Mux3/5
  In12/1 -> Gen. Heat (MW)/1
  [BattPow] -> Battery storage system/1
  [BatteryEnergy] -> Battery storage system/2
  [BatterySOC] -> Battery storage system/3
  [HeatStorageSOC] -> Heat Storage system/3
  [TotalElectPow] -> Mux6/2
  Mux6/1 -> FC power - Cons. elect power/1
  Product1/1 -> Auxiliary electricity power/1
  [PropCurrent] -> Product/1
  [BusVoltage] -> Product1/2
  [BusVoltage] -> Product/2
  [PropPower] -> Propulsion electrical power/2
  [BusVoltage] -> Bus voltage/1
  [AuxElPow] -> Auxiliary electricity power/2
  [FCBusCurrent] -> Product4/1
  [AuxElCurrent] -> Product1/1
  [BusVoltage] -> Product4/2
  Product/1 -> Propulsion electrical power/1
  Product4/1 -> Mux6/1
  Divide1/1 -> [BatterySOC]
  Divide/1 -> Divide1/1, [BatteryEnergy]
  Power to energy [W*s]/1 -> Divide/1
  Mux7/1 -> Currents/1
  [FCBusCurrent] -> Mux7/1
  [BattCurrent] -> Product5/1
  Constant1/1 -> Divide1/2
  Product5/1 -> [BattPow]
  [BattCurrent] -> Mux7/2
  [BusCurrent] -> Mux7/3
  Constant/1 -> Divide/2
  [BattPow] -> Power to energy [W*s]/1
  [BusVoltage] -> Product5/2

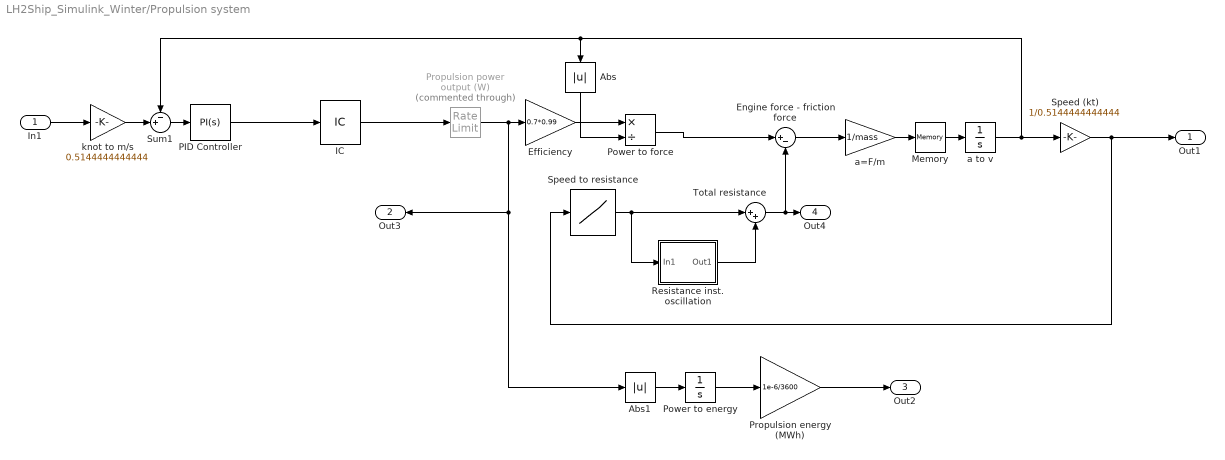
== system LH2Ship_Simulink_Winter/Propulsion system ==
  In1 : Inport
  Abs : Abs
  Abs1 : Abs
  Efficiency : Gain  Gain=0.7*0.99
  Engine force - friction force : Sum  Inputs=|+-
  IC : InitialCondition  Value=2e7
  Memory : Memory  InitialCondition=16.66*0.51444444
  PID Controller : simulink/Continuous/PID Controller  Controller=PI  Form=Parallel  TimeDomain=Continuous-time  SampleTime=-1  IntegratorMethod=Forward Euler  FilterMethod=Forward Euler  ControllerParametersSource=internal  P=9967066.66982428  I=15836.3521855852  D=676782585.714132  UseFilter=on  N=0.00702265439594147  TunerSelectOption=Transfer Function Based (PID Tuner App)  InitialConditionSource=internal  InitialConditionForIntegrator=2e7  InitialConditionForFilter=0  DifferentiatorICPrevScaledInput=0  ExternalReset=none  TrackingMode=off  Kt=1  LimitOutput=on  UpperSaturationLimit=60000000  LowerSaturationLimit=-60000000  LinearizeAsGain=off  AntiWindupMode=clamping  Kb=1  POutMin=[]  POutMax=[]  IOutMin=[]  IOutMax=[]  DOutMin=[]  DOutMax=[]  NOutMin=[]  NOutMax=[]  SumOutMin=[]  SumOutMax=[]  SaturationOutMin=[]  SaturationOutMax=[]  PParamMin=[]  PParamMax=[]  IParamMin=[]  IParamMax=[]  DParamMin=[]  DParamMax=[]  NParamMin=[]  NParamMax=[]  KbParamMin=[]  KbParamMax=[]  KtParamMin=[]  KtParamMax=[]  KbOutMin=[]  KbOutMax=[]  KtOutMin=[]  KtOutMax=[]  IntegratorOutMin=[]  IntegratorOutMax=[]  FilterOutMin=[]  FilterOutMax=[]  SumI1OutMin=[]  SumI1OutMax=[]  SumI2OutMin=[]  SumI2OutMax=[]  SumI3OutMin=[]  SumI3OutMax=[]  SumI4OutMin=[]  SumI4OutMax=[]  SumDOutMin=[]  SumDOutMax=[]  DifferentiatorOutMin=[]  DifferentiatorOutMax=[]  FilterDiffOutCoefMin=[]  FilterDiffOutCoefMax=[]  ReciprocalOutMin=[]  ReciprocalOutMax=[]  SumDenOutMin=[]  SumDenOutMax=[]  SumNumOutMin=[]  SumNumOutMax=[]  DivideOutMin=[]  DivideOutMax=[]  IntegratorContinuousStateAttributes=''  IntegratorStateMustResolveToSignalObject=off  IntegratorRTWStateStorageClass=Auto  FilterContinuousStateAttributes=''  FilterStateMustResolveToSignalObject=off  FilterRTWStateStorageClass=Auto  ParallelPVariant=InternalParameters  IdealPVariant=Disabled  IVariant=InternalParameters  DVariant=Disabled  IntegratorVariant=Continuous  SatVariant=Enabled  AWVariant=ContClampingParallel  PCopyVariant=Disabled  TRVariant=Disabled  FdbkBlocksVariant=Forward  IdealPFdbkVariant=Disabled  SatFdbkVariant=Disabled  DerivativeFilterVariant=Disabled  NVariant=Disabled  NCopyVariant=Disabled_SignalSpec  FilterICVariant=Disabled  IntegratorICVariant=InternalICs  ExternalResetVariant=Disabled  TRSumVariant=Passthrough  SumFdbkVariant=Disabled  SumVariant=Sum_PI
  Power to energy : Integrator  LowerSaturationLimit=0
  Power to force : Product  Inputs=*/
  Propulsion power output (W) : RateLimiter  Commented=through  RisingSlewLimit=1000000  FallingSlewLimit=-inf  SampleTimeMode=inherited
  Propulsion energy (MWh) : Gain  Gain=1e-6/3600
  Resistance inst. oscillation : Subsystem
  Speed (kt) : Gain  Gain=1/0.5144444444444
  Speed to resistance : Lookup  InputValues=v  Table=Rt
  Sum1 : Sum  Inputs=-+|
  Total resistance : Sum  Inputs=|++
  a to v : Integrator  InitialCondition=16.66*0.51444444  LowerSaturationLimit=0
  a=F/m : Gain  Gain=1/mass
  knot to m/s : Gain  Gain=0.5144444444444
  Out1 : Outport
  Out3 : Outport  Port=2
  Out2 : Outport  Port=3
  Out4 : Outport  Port=4
  wires:
  Speed to resistance/1 -> Resistance inst. oscillation/1(In1), Total resistance/1
  Propulsion energy (MWh)/1 -> Out2/1
  Resistance inst. oscillation/1(Out1) -> Total resistance/2
  a to v/1 -> Abs/1, Sum1/1, Speed (kt)/1
  Abs/1 -> Power to force/2
  Total resistance/1 -> Out4/1, Engine force - friction force/2
  Sum1/1 -> PID Controller/1
  knot to m/s/1 -> Sum1/2
  Power to energy/1 -> Propulsion energy (MWh)/1
  Abs1/1 -> Power to energy/1
  PID Controller/1 -> IC/1
  Speed (kt)/1 -> Speed to resistance/1, Out1/1
  Propulsion power output (W)/1 -> Out3/1, Abs1/1, Efficiency/1
  In1/1 -> knot to m/s/1
  Power to force/1 -> Engine force - friction force/1
  Engine force - friction force/1 -> a=F/m/1
  Efficiency/1 -> Power to force/1
  IC/1 -> Propulsion power output (W)/1
  a=F/m/1 -> Memory/1
  Memory/1 -> a to v/1

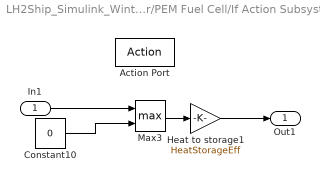
== system LH2Ship_Simulink_Winter/PEM Fuel Cell/If Action Subsystem ==
  In1 : Inport
  Action Port : ActionPort  ActionType=then
  Constant10 : Constant  Value=0
  Heat to storage1 : Gain  Gain=HeatStorageEff
  Max3 : MinMax  Function=max  Inputs=2
  Out1 : Outport
  wires:
  Constant10/1 -> Max3/2
  In1/1 -> Max3/1
  Max3/1 -> Heat to storage1/1
  Heat to storage1/1 -> Out1/1

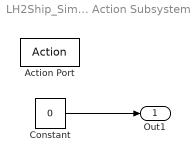
== system LH2Ship_Simulink_Winter/PEM Fuel Cell/If Action Subsystem1 ==
  Action Port : ActionPort  ActionType=else
  Constant : Constant  Value=0
  Out1 : Outport
  wires:
  Constant/1 -> Out1/1

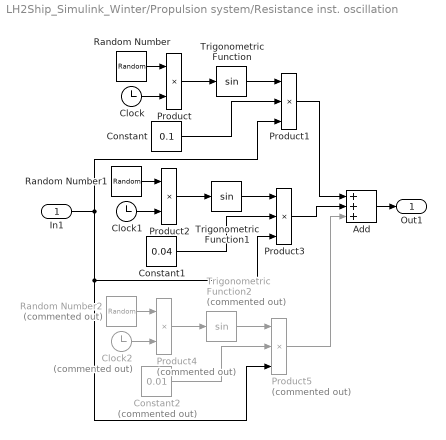
== system LH2Ship_Simulink_Winter/Propulsion system/Resistance inst. oscillation ==
  In1 : Inport
  Add : Sum  Inputs=3
  Clock : Clock
  Clock1 : Clock
  Clock2 : Clock  Commented=on
  Constant : Constant  Value=0.1
  Constant1 : Constant  Value=0.04
  Constant2 : Constant  Commented=on  Value=0.01
  Product : Product
  Product1 : Product  Inputs=3
  Product2 : Product
  Product3 : Product  Inputs=3
  Product4 : Product  Commented=on
  Product5 : Product  Commented=on  Inputs=3
  Random Number : RandomNumber  Mean=pi/1000000  Variance=0.00000005  Seed=0.00005  SampleTime=100
  Random Number1 : RandomNumber  Mean=pi/6  Variance=0.5  Seed=0.3  SampleTime=200
  Random Number2 : RandomNumber  Commented=on  Mean=pi  Variance=3  Seed=3  SampleTime=10
  Trigonometric Function : Trigonometry
  Trigonometric Function1 : Trigonometry
  Trigonometric Function2 : Trigonometry  Commented=on
  Out1 : Outport
  wires:
  Clock2/1 -> Product4/2
  Clock/1 -> Product/2
  Product4/1 -> Trigonometric Function2/1
  Constant/1 -> Product1/2
  Clock1/1 -> Product2/2
  Product/1 -> Trigonometric Function/1
  In1/1 -> Product5/3, Product3/3, Product1/3
  Product5/1 -> Add/3
  Product1/1 -> Add/1
  Trigonometric Function1/1 -> Product3/1
  Constant1/1 -> Product3/2
  Product2/1 -> Trigonometric Function1/1
  Random Number1/1 -> Product2/1
  Constant2/1 -> Product5/2
  Trigonometric Function/1 -> Product1/1
  Random Number/1 -> Product/1
  Add/1 -> Out1/1
  Product3/1 -> Add/2
  Trigonometric Function2/1 -> Product5/1
  Random Number2/1 -> Product4/1
